simulink model "ActiveSupensionNonlinear"  (R2019b)
settings: Solver=ode45  StartTime=0.0  StopTime=10  RelTol=1e-3  EnableMultiTasking=on
values from neighbouring files (symbols this model uses):
  b = 1000    [parameters.m]    (also in run_FLC_simulation.m)
  k1 = 16000    [parameters.m]
  k2 = 190000    [parameters.m]    (also in run_FLC_simulation.m)
  k_nl = 50000    [TS_simulation.m]    (also in parameters.m = 500; quarter_car_sat_v4.m = min(ks + alpha*x1^2, k1_max); run_FLC_simulation.m)
  mb = 285    [H.m]    (also in LMI_results.mat = 300; parameters.m = 300; plot_comparison.m = 300; run_FLC_simulation.m = 300)
  mw = 60    [H.m]    (also in LMI_results.mat; parameters.m; plot_comparison.m; run_FLC_simulation.m)
settings Model: Creator=MLRida  LastModifiedBy=admin
settings DataIOCC: LimitDataPoints=on  SaveFormat=Array  ReturnWorkspaceOutputs=off
settings OptimizationCC: LifeSpan=inf
settings DebuggingCC: SolverPrmCheckMsg=warning  SFUnexpectedBacktrackingDiag=warning  SFNoUnconditionalDefaultTransitionDiag=warning  SFExecutionAtInitializationDiag=none  ArithmeticOperatorsInVariantConditions=warning
settings HardwareCC: ProdBitPerPointer=32  ProdBitPerSizeT=32  ProdBitPerPtrDiffT=32  ProdLargestAtomicFloat=None  ProdIntDivRoundTo=Undefined  ProdEndianess=Unspecified  ProdWordSize=32  ProdHWDeviceType=32-bit Generic
settings ModelReferenceCC: PropagateSignalLabelsOutOfModel=off
settings SFSimCC: SimUseLocalCustomCode=off  CustomCodeUndefinedFunction=UseInterfaceOnly
settings RTWCC: RTWUseLocalCustomCode=off
settings CodeAppCC: StateflowObjectComments=on
settings GRTTargetCC: TargetLangStandard=C89/C90 (ANSI)  GeneratePreprocessorConditionals=Disable all
settings ConfigComp: CovMetricSettings=dw  CovHtmlReporting=on  CovSaveCumulativeToWorkspaceVar=on  CovSaveSingleToWorkspaceVar=on  CovExternalEMLEnable=off  CovSFcnEnable=off

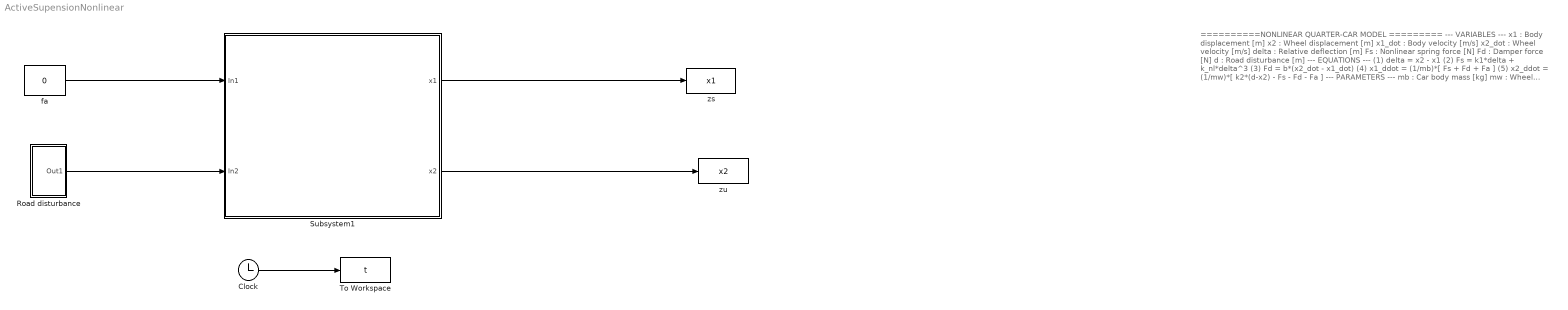
== system ActiveSupensionNonlinear ==
  note: ==========NONLINEAR QUARTER-CAR MODEL =========
      |
      | --- VARIABLES ---
      | x1 : Body displacement [m]
      | x2 : Wheel displacement [m]
      | x1_dot : Body velocity [m/s]
      | x2_dot : Wheel velocity [m/s]
      | delta : Relative deflection [m]
      | Fs : Nonlinear spring force [N]
      | Fd : Damper force [N]
      | d : Road disturbance [m]
      |
      | --- EQUATIONS ---
      | (1) delta = x2 - x1
      | (2) Fs = k1*delta + k_nl*delta^3
      | (3) Fd = b*(x2_dot - x1_dot)
      | (4) x1_ddot = (1/mb)*[ Fs + Fd + Fa ]
      | (5) x2_ddot = (1/mw)*[ k2*(d-x2) - Fs - Fd - Fa ]
      |
      | --- PARAMETERS ---
      | mb : Car body mass [kg]
      | mw : Wheel mass [kg]
      | k1 : Linear spring stiffness [N/m]
      | k_nl : Cubic nonlinear coefficient [N/m^3]
      | b : Damper coefficient [N.s/m]
      | k2 : Tyre stiffness [N/m]
      | Fa : Active actuator force [N]
      |
      | --- STATES ---
      | x = [ x1 ; x1_dot ; x2 ; x2_dot ]
      |
      | --- INPUT ---
      | u = [ Fa ; d_road ]
  Clock : Clock
  Road disturbance : Subsystem
  Subsystem1 : Subsystem
  To Workspace : ToWorkspace  VariableName=t  SampleTime=0.001
  fa : Constant  Value=0
  zs : ToWorkspace  VariableName=x1  SampleTime=0.001
  zu : ToWorkspace  VariableName=x2  SampleTime=0.001
  wires:
  Clock/1 -> To Workspace/1
  fa/1 -> Subsystem1/1(In1)
  Road disturbance/1(Out1) -> Subsystem1/2(In2)
  Subsystem1/1(x1) -> zs/1
  Subsystem1/2(x2) -> zu/1

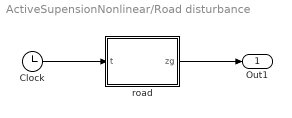
== system ActiveSupensionNonlinear/Road disturbance ==
  Clock : Clock
  "road " : MATLAB Function  TreatAsAtomicUnit=on
  Out1 : Outport
  wires:
  "road "/1(zg) -> Out1/1
  Clock/1 -> "road "/1(t)

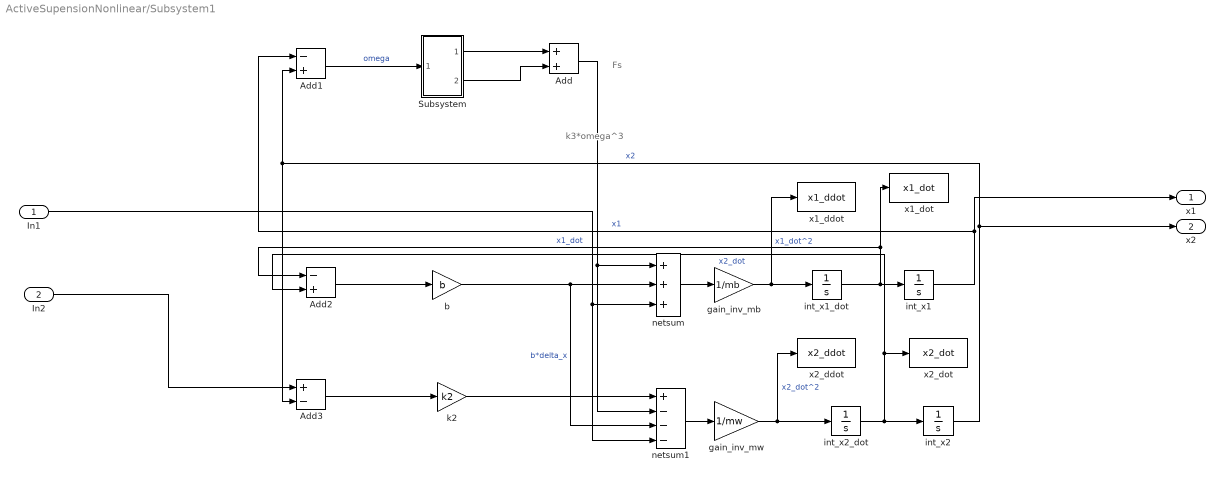
== system ActiveSupensionNonlinear/Subsystem1 ==
  note: k3*omega^3
  note: Fs
  In1 : Inport
  In2 : Inport  Port=2
  Add : Sum
  Add1 : Sum  Inputs=-+
  Add2 : Sum  Inputs=-+
  Add3 : Sum  Inputs=+-
  Subsystem : Subsystem
  b : Gain  Gain=b
  gain_inv_mb : Gain  Gain=1/mb
  "gain_inv_mw " : Gain  Gain=1/mw
  int_x1 : Integrator  InitialCondition=0.001
  "int_x1_dot " : Integrator  InitialCondition=0.001
  int_x2 : Integrator  InitialCondition=0.001
  "int_x2_dot " : Integrator  InitialCondition=0.001
  "k2 " : Gain  Gain=k2
  netsum : Sum  Inputs=+++  SaturateOnIntegerOverflow=on  InputSameDT=on  OutDataTypeStr=Inherit: Same as first input
  netsum1 : Sum  Inputs=+---  SaturateOnIntegerOverflow=on  InputSameDT=on  OutDataTypeStr=Inherit: Same as first input
  x1_ddot : ToWorkspace  VariableName=x1_ddot  SampleTime=0.001
  x1_dot : ToWorkspace  VariableName=x1_dot  SampleTime=0.001
  x2_ddot : ToWorkspace  VariableName=x2_ddot  SampleTime=0.001
  x2_dot : ToWorkspace  VariableName=x2_dot  SampleTime=0.001
  x1 : Outport
  x2 : Outport  Port=2
  wires:
  Subsystem/1(Out1) -> Add/1
  gain_inv_mb/1 -> x1_ddot/1, "int_x1_dot "/1  "x1_dot^2"
  Add/1 -> netsum/1, netsum1/2
  netsum1/1 -> "gain_inv_mw "/1
  Add1/1 -> Subsystem/1(In1)  "omega"
  In1/1 -> netsum1/4, netsum/3
  "gain_inv_mw "/1 -> "int_x2_dot "/1, x2_ddot/1  "x2_dot^2"
  Add2/1 -> b/1
  b/1 -> netsum1/3, netsum/2  "b*delta_x"
  In2/1 -> Add3/1
  int_x2/1 -> x2/1, Add3/2, Add1/2  "x2"
  int_x1/1 -> x1/1, Add1/1  "x1"
  Add3/1 -> "k2 "/1
  Subsystem/2(Out2) -> Add/2
  "k2 "/1 -> netsum1/1
  netsum/1 -> gain_inv_mb/1
  "int_x2_dot "/1 -> x2_dot/1, Add2/2, int_x2/1  "x2_dot"
  "int_x1_dot "/1 -> x1_dot/1, Add2/1, int_x1/1  "x1_dot"

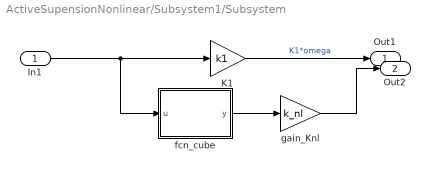
== system ActiveSupensionNonlinear/Subsystem1/Subsystem ==
  In1 : Inport
  "K1 " : Gain  Gain=k1
  "fcn_cube " : MATLAB Function  TreatAsAtomicUnit=on
  "gain_Knl " : Gain  Gain=k_nl
  Out1 : Outport
  Out2 : Outport  Port=2
  wires:
  "fcn_cube "/1(y) -> "gain_Knl "/1
  "gain_Knl "/1 -> Out2/1
  In1/1 -> "fcn_cube "/1(u), "K1 "/1
  "K1 "/1 -> Out1/1  "K1*omega"

== matlab function ActiveSupensionNonlinear/Subsystem1/Subsystem/fcn_cube  ==
  data: u input; y output
function y = fcn_cube(u)
% ========================================================
%  EXTERNAL FUNCTION: Cubic Nonlinear Term
%  --------------------------------------------------------
%  Input  : u  --> delta = x2 - x1  (relative deflection)
%  Output : y  --> u^3
% ========================================================

    y = u.^3;

end

== matlab function ActiveSupensionNonlinear/Road disturbance/road  ==
  data: t input; zg output
function zg = road_disturbance(t)

% -------------------------------
% Parameters
% -------------------------------
h = 0.04;     % bump height (m)
T = 0.5;      % bump duration (s)
t0 = 1;       % start time (s)

% -------------------------------
% Half-sine bump
% -------------------------------
if t >= t0 && t <= t0 + T
    zg = (h/2) * (1 - cos(2*pi*(t - t0)/T));
else
    zg = 0;
end

end
